simulink library "FlightInstruments"  (R2023a)
settings: Solver=VariableStepAuto  StartTime=0.0  StopTime=10.0  RelTol=1e-3
PostLoadFcn:
  | set_param(gcs,'Location',get(0,'ScreenSize'));
settings Model: Creator=LSV-PC0  LastModifiedBy=LSV-PC0

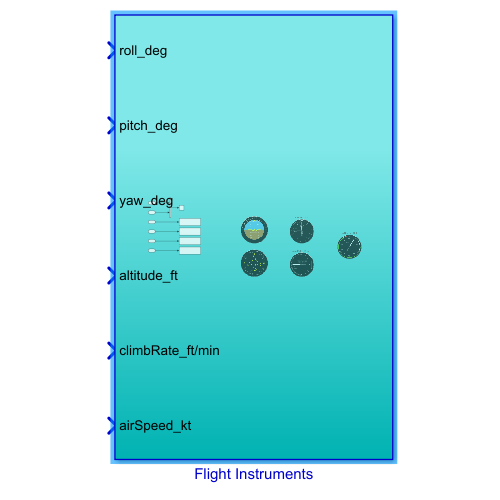
[thumbnail: Simulink's stored preview of the top-level diagram]
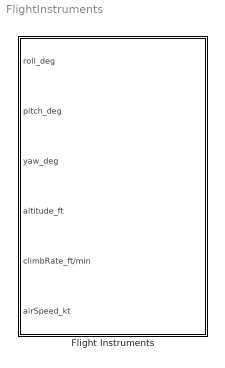
== system FlightInstruments ==
  Flight Instruments : Subsystem

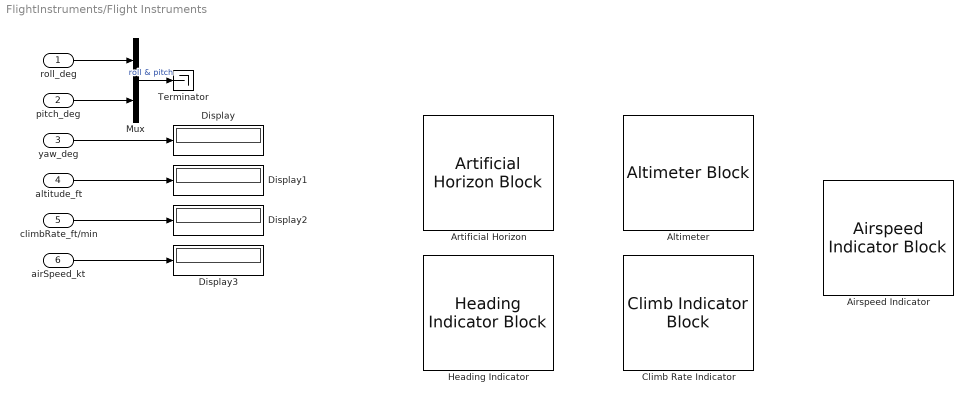
== system FlightInstruments/Flight Instruments ==
  roll_deg : Inport
  pitch_deg : Inport  Port=2
  yaw_deg : Inport  Port=3
  altitude_ft : Inport  Port=4
  climbRate_ft/min : Inport  Port=5
  airSpeed_kt : Inport  Port=6
  Airspeed Indicator : AirspeedIndicatorBlock
  Altimeter : AltimeterBlock
  Artificial Horizon : ArtificialHorizonBlock  LabelPosition=Hide
  Climb Rate Indicator : ClimbIndicatorBlock
  Display{,1..3} (4 alike) : Display
  Heading Indicator : HeadingIndicatorBlock  LabelPosition=Hide
  Mux : Mux  Inputs=2
  Terminator : Terminator
  wires:
  Mux/1 -> Terminator/1  "roll & pitch"
  yaw_deg/1 -> Display/1
  climbRate_ft/min/1 -> Display2/1
  airSpeed_kt/1 -> Display3/1
  roll_deg/1 -> Mux/1
  altitude_ft/1 -> Display1/1
  pitch_deg/1 -> Mux/2
